simulink model "mariner_NNcont"  (R2018b)
settings: Solver=FixedStepAuto  StartTime=0.0  StopTime=600  FixedStep=0.1  RelTol=1e-3
libraries: neural x75, simulink x1
(part 3 of 3)

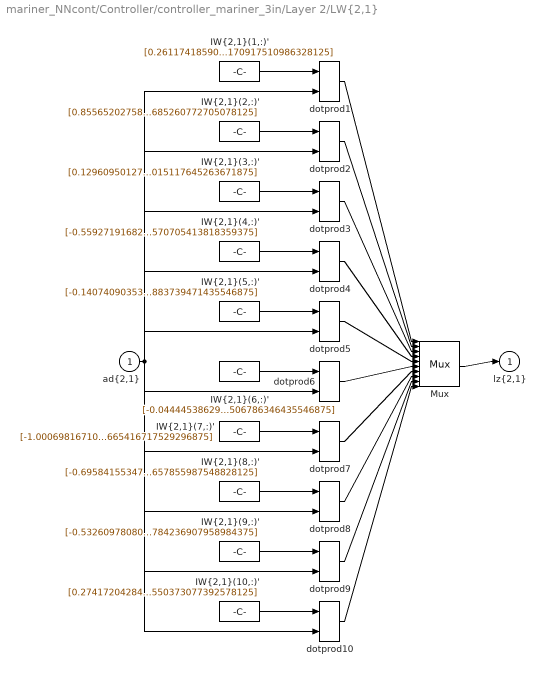
== system mariner_NNcont/Controller/controller_mariner_3in/Layer 2/LW{2,1} ==
  "ad{2,1}" : Inport  PortDimensions=10
      mask Display: e = 0.06;c1 = [120 230 180]/255;c2 = ([120 230 180]+0)/(256+128);c3 = ([120 230 180]+128)/(256+128);patch([0 1 1 0],[0 0 1 1],c1);patch([0 1 1 1-e 1-e 0+e],[0 0 1 1-e 0+e 0+e],c2);patch([0 0 1 1-e 0+e 0+e],[0 1 1 1-e 1-e 0+e],c3);plot([0 1 1 0 0],[0 0 1 1 0]);
  "IW{2,1}(1,:)'" : Constant  Value=[0.261174185904248068457178533208207227289676666259765625;-0.003283003051929162842414999801121666678227484226226806640625;0.21894073243983969145887158447294495999813079833984375;0.1719351505134853186351762133199372328817844390869140625;-0.79630547007300067630097828441648744046688079833984375;-0.444574661776908464094759665385936386883258819580078125;0.906078837819613180926126005942933261394500732421875;-0.5775547854832592253870870990795083343982696533203125;0.3749229122076920273087807800038717687129974365234375;-0.91313009543488476982275869886507280170917510986328125]
      mask Display: e = 0.06;c1 = [120 150 230]/255;c2 = ([120 150 230]+0)/383;c3 = ([120 150 230]+128)/383;patch([0 1 1 0],[0 0 1 1],c1);patch([0 1 1 1-e 1-e 0+e],[0 0 1 1-e 0+e 0+e],c2);patch([0 0 1 1-e 0+e 0+e],[0 1 1 1-e 1-e 0+e],c3);plot([0 1 1 0 0],[0 0 1 1 0]);disp('weights');
  "IW{2,1}(10,:)'" : Constant  Value=[0.2741720428489411442996015466633252799510955810546875;-0.331267567288568820504934819837217219173908233642578125;0.08501797064077308563323498447061865590512752532958984375;-0.13802843406108300516876852270797826349735260009765625;-0.66775067067659055197736961417831480503082275390625;0.65274589167754093477213928053970448672771453857421875;0.60325942316056535563717488912516273558139801025390625;0.76541902649870774411056117969565093517303466796875;-0.302998665532592859062077650378341786563396453857421875;1.014969024792983010030411605839617550373077392578125]
      mask Display: e = 0.06;c1 = [120 150 230]/255;c2 = ([120 150 230]+0)/383;c3 = ([120 150 230]+128)/383;patch([0 1 1 0],[0 0 1 1],c1);patch([0 1 1 1-e 1-e 0+e],[0 0 1 1-e 0+e 0+e],c2);patch([0 0 1 1-e 0+e 0+e],[0 1 1 1-e 1-e 0+e],c3);plot([0 1 1 0 0],[0 0 1 1 0]);disp('weights');
  "IW{2,1}(2,:)'" : Constant  Value=[0.85565202758614222755539913123357109725475311279296875;-0.283056952913707082775118806239333935081958770751953125;-0.2258338801321223832108131546192453242838382720947265625;0.77075660919109056923304024167009629309177398681640625;-0.1294753607797942962509551989569445140659809112548828125;0.152371280591739377552329415266285650432109832763671875;0.0399229534231867744242805429166764952242374420166015625;-0.75982138249167163746022879422525875270366668701171875;-0.80225466104966314251356607201159931719303131103515625;-0.62172867186234548331214000427280552685260772705078125]
      mask Display: e = 0.06;c1 = [120 150 230]/255;c2 = ([120 150 230]+0)/383;c3 = ([120 150 230]+128)/383;patch([0 1 1 0],[0 0 1 1],c1);patch([0 1 1 1-e 1-e 0+e],[0 0 1 1-e 0+e 0+e],c2);patch([0 0 1 1-e 0+e 0+e],[0 1 1 1-e 1-e 0+e],c3);plot([0 1 1 0 0],[0 0 1 1 0]);disp('weights');
  "IW{2,1}(3,:)'" : Constant  Value=[0.1296095012754385766839959615026600658893585205078125;-0.94480799299970896765188399513135664165019989013671875;-0.4301375963937488222654792480170726776123046875;0.459664837526012615143145012552849948406219482421875;0.1934938854259011520309030629505286924540996551513671875;0.303590659028730447399624381432658992707729339599609375;0.0250667137529580787147498455169625231064856052398681640625;-0.7718185476396290933820409918553195893764495849609375;-0.7919589744969688371867277965066023170948028564453125;-0.6689404878056404157860015402548015117645263671875]
      mask Display: e = 0.06;c1 = [120 150 230]/255;c2 = ([120 150 230]+0)/383;c3 = ([120 150 230]+128)/383;patch([0 1 1 0],[0 0 1 1],c1);patch([0 1 1 1-e 1-e 0+e],[0 0 1 1-e 0+e 0+e],c2);patch([0 0 1 1-e 0+e 0+e],[0 1 1 1-e 1-e 0+e],c3);plot([0 1 1 0 0],[0 0 1 1 0]);disp('weights');
  "IW{2,1}(4,:)'" : Constant  Value=[-0.5592719168271766960742752416990697383880615234375;-0.63972010553606384331004619525629095733165740966796875;0.86712354687803727681938426030683331191539764404296875;-0.60202632961644775289045128374709747731685638427734375;0.04675818126060522772480254616311867721378803253173828125;-0.6845715113228525439126315177418291568756103515625;0.1082908321127431239272453922239947132766246795654296875;-0.2114272144397531250081812004282255657017230987548828125;0.1653939942029022114322600600644364021718502044677734375;0.85845774340393798951254211715422570705413818359375]
      mask Display: e = 0.06;c1 = [120 150 230]/255;c2 = ([120 150 230]+0)/383;c3 = ([120 150 230]+128)/383;patch([0 1 1 0],[0 0 1 1],c1);patch([0 1 1 1-e 1-e 0+e],[0 0 1 1-e 0+e 0+e],c2);patch([0 0 1 1-e 0+e 0+e],[0 1 1 1-e 1-e 0+e],c3);plot([0 1 1 0 0],[0 0 1 1 0]);disp('weights');
  "IW{2,1}(5,:)'" : Constant  Value=[-0.14074090353561474753263382808654569089412689208984375;-0.1582177881605986990987133822272880934178829193115234375;0.76789061341721709386121119678136892616748809814453125;-0.64243771524855175503176951679051853716373443603515625;0.6982728307682517510102115920744836330413818359375;0.0301621836322126524176923112463555298745632171630859375;0.34029705620992156678283890869352035224437713623046875;0.771669895262477201214323940803296864032745361328125;0.430887484942656551201167758335941471159458160400390625;0.82439589529222967456689730170182883739471435546875]
      mask Display: e = 0.06;c1 = [120 150 230]/255;c2 = ([120 150 230]+0)/383;c3 = ([120 150 230]+128)/383;patch([0 1 1 0],[0 0 1 1],c1);patch([0 1 1 1-e 1-e 0+e],[0 0 1 1-e 0+e 0+e],c2);patch([0 0 1 1-e 0+e 0+e],[0 1 1 1-e 1-e 0+e],c3);plot([0 1 1 0 0],[0 0 1 1 0]);disp('weights');
  "IW{2,1}(6,:)'" : Constant  Value=[-0.04444538629282100694606327806468470953404903411865234375;0.1633126529035742457995894483246956951916217803955078125;0.93328352617765852894393674432649277150630950927734375;0.1312587739791350738283171040166052989661693572998046875;-0.88766423248751002983425451020593754947185516357421875;-0.00598139511896102205046332755955518223345279693603515625;-0.86611856253597918620101836495450697839260101318359375;-0.785777466061251761431094564613886177539825439453125;-0.10379331601532486295536017451013321988284587860107421875;-0.1520954521603174736110730691507342271506786346435546875]
      mask Display: e = 0.06;c1 = [120 150 230]/255;c2 = ([120 150 230]+0)/383;c3 = ([120 150 230]+128)/383;patch([0 1 1 0],[0 0 1 1],c1);patch([0 1 1 1-e 1-e 0+e],[0 0 1 1-e 0+e 0+e],c2);patch([0 0 1 1-e 0+e 0+e],[0 1 1 1-e 1-e 0+e],c3);plot([0 1 1 0 0],[0 0 1 1 0]);disp('weights');
  "IW{2,1}(7,:)'" : Constant  Value=[-1.0006981671063766015095097827725112438201904296875;0.60941030927903039327020451310090720653533935546875;-0.02375081956900626511952623332035727798938751220703125;-0.155539049648913241252756733956630341708660125732421875;-0.87176861100853397790189092120272107422351837158203125;0.2349462648057879798901836920776986517012119293212890625;-0.78217384326468419875055815282394178211688995361328125;-0.4284269793998471964613372620078735053539276123046875;-0.25720118636501931863591607907437719404697418212890625;0.17938257051239059336467107641510665416717529296875]
      mask Display: e = 0.06;c1 = [120 150 230]/255;c2 = ([120 150 230]+0)/383;c3 = ([120 150 230]+128)/383;patch([0 1 1 0],[0 0 1 1],c1);patch([0 1 1 1-e 1-e 0+e],[0 0 1 1-e 0+e 0+e],c2);patch([0 0 1 1-e 0+e 0+e],[0 1 1 1-e 1-e 0+e],c3);plot([0 1 1 0 0],[0 0 1 1 0]);disp('weights');
  "IW{2,1}(8,:)'" : Constant  Value=[-0.69584155347007980996210108060040511190891265869140625;0.75309159965000371794729971952619962394237518310546875;-0.75210268731275908837830002084956504404544830322265625;0.71218767580268649286523441332974471151828765869140625;0.69666567607896545677448330025072209537029266357421875;0.106029491219146565494924061567871831357479095458984375;0.293510496575862589452299289405345916748046875;-0.276039693004178798840797526281676255166530609130859375;-0.10816770394463266768969589293192257173359394073486328125;0.652295803383552641463438703794963657855987548828125]
      mask Display: e = 0.06;c1 = [120 150 230]/255;c2 = ([120 150 230]+0)/383;c3 = ([120 150 230]+128)/383;patch([0 1 1 0],[0 0 1 1],c1);patch([0 1 1 1-e 1-e 0+e],[0 0 1 1-e 0+e 0+e],c2);patch([0 0 1 1-e 0+e 0+e],[0 1 1 1-e 1-e 0+e],c3);plot([0 1 1 0 0],[0 0 1 1 0]);disp('weights');
  "IW{2,1}(9,:)'" : Constant  Value=[-0.53260978080398280187779391781077720224857330322265625;0.7797854193828011037936676075332798063755035400390625;1.0309904985328952609080488400650210678577423095703125;0.2090678564933573790884935306166880764067173004150390625;0.422970982361082270539753835691954009234905242919921875;-0.25386727615109305755680679794750176370143890380859375;0.64856644515765704550602777089807204902172088623046875;0.0214787671671146894458725995491477078758180141448974609375;0.402204635550879763261633570436970330774784088134765625;-0.53082955432786516070109428255818784236907958984375]
      mask Display: e = 0.06;c1 = [120 150 230]/255;c2 = ([120 150 230]+0)/383;c3 = ([120 150 230]+128)/383;patch([0 1 1 0],[0 0 1 1],c1);patch([0 1 1 1-e 1-e 0+e],[0 0 1 1-e 0+e 0+e],c2);patch([0 0 1 1-e 0+e 0+e],[0 1 1 1-e 1-e 0+e],c3);plot([0 1 1 0 0],[0 0 1 1 0]);disp('weights');
  Mux : Mux  Inputs=10
      mask Display: e = 0.06;c1 = [120 150 230]/255;c2 = ([120 150 230]+0)/383;c3 = ([120 150 230]+128)/383;patch([0 1 1 0],[0 0 1 1],c1);patch([0 1 1 1-e 1-e 0+e],[0 0 1 1-e 0+e 0+e],c2);patch([0 0 1 1-e 0+e 0+e],[0 1 1 1-e 1-e 0+e],c3);plot([0 1 1 0 0],[0 0 1 1 0]);disp('Mux');
  dotprod{1..10} (10 alike) : neural/Weight Functions/dotprod
  "lz{2,1}" : Outport
      mask Display: e = 0.06;c1 = [120 230 180]/255;c2 = ([120 230 180]+0)/(256+128);c3 = ([120 230 180]+128)/(256+128);patch([0 1 1 0],[0 0 1 1],c1);patch([0 1 1 1-e 1-e 0+e],[0 0 1 1-e 0+e 0+e],c2);patch([0 0 1 1-e 0+e 0+e],[0 1 1 1-e 1-e 0+e],c3);plot([0 1 1 0 0],[0 0 1 1 0]);
  wires:
  Mux/1 -> "lz{2,1}"/1
  dotprod10/1 -> Mux/10
  "IW{2,1}(10,:)'"/1 -> dotprod10/1
  dotprod9/1 -> Mux/9
  "IW{2,1}(9,:)'"/1 -> dotprod9/1
  dotprod8/1 -> Mux/8
  "IW{2,1}(8,:)'"/1 -> dotprod8/1
  dotprod7/1 -> Mux/7
  "IW{2,1}(7,:)'"/1 -> dotprod7/1
  dotprod6/1 -> Mux/6
  "IW{2,1}(6,:)'"/1 -> dotprod6/1
  dotprod5/1 -> Mux/5
  "IW{2,1}(5,:)'"/1 -> dotprod5/1
  dotprod4/1 -> Mux/4
  "IW{2,1}(4,:)'"/1 -> dotprod4/1
  dotprod3/1 -> Mux/3
  "IW{2,1}(3,:)'"/1 -> dotprod3/1
  dotprod2/1 -> Mux/2
  "IW{2,1}(2,:)'"/1 -> dotprod2/1
  dotprod1/1 -> Mux/1
  "ad{2,1}"/1 -> dotprod10/2, dotprod9/2, dotprod8/2, dotprod7/2, dotprod6/2, dotprod5/2, dotprod4/2, dotprod3/2, dotprod2/2, dotprod1/2
  "IW{2,1}(1,:)'"/1 -> dotprod1/1

== system mariner_NNcont/Controller/controller_mariner_3in/Layer 3/Delays 1 ==
  "p{3}" : Inport  PortDimensions=10
      mask Display: e = 0.06;c1 = [120 230 180]/255;c2 = ([120 230 180]+0)/(256+128);c3 = ([120 230 180]+128)/(256+128);patch([0 1 1 0],[0 0 1 1],c1);patch([0 1 1 1-e 1-e 0+e],[0 0 1 1-e 0+e 0+e],c2);patch([0 0 1 1-e 0+e 0+e],[0 1 1 1-e 1-e 0+e],c3);plot([0 1 1 0 0],[0 0 1 1 0]);
  mux : Mux  Inputs=1
      mask Display: e = 0.06;c1 = [120 150 230]/255;c2 = ([120 150 230]+0)/383;c3 = ([120 150 230]+128)/383;patch([0 1 1 0],[0 0 1 1],c1);patch([0 1 1 1-e 1-e 0+e],[0 0 1 1-e 0+e 0+e],c2);patch([0 0 1 1-e 0+e 0+e],[0 1 1 1-e 1-e 0+e],c3);plot([0 1 1 0 0],[0 0 1 1 0]);disp('Mux')
  "pd{3,2}" : Outport
      mask Display: e = 0.06;c1 = [120 230 180]/255;c2 = ([120 230 180]+0)/(256+128);c3 = ([120 230 180]+128)/(256+128);patch([0 1 1 0],[0 0 1 1],c1);patch([0 1 1 1-e 1-e 0+e],[0 0 1 1-e 0+e 0+e],c2);patch([0 0 1 1-e 0+e 0+e],[0 1 1 1-e 1-e 0+e],c3);plot([0 1 1 0 0],[0 0 1 1 0]);
  wires:
  mux/1 -> "pd{3,2}"/1
  "p{3}"/1 -> mux/1

== system mariner_NNcont/Controller/controller_mariner_3in/Layer 3/LW{3,2} ==
  "ad{3,2}" : Inport  PortDimensions=10
      mask Display: e = 0.06;c1 = [120 230 180]/255;c2 = ([120 230 180]+0)/(256+128);c3 = ([120 230 180]+128)/(256+128);patch([0 1 1 0],[0 0 1 1],c1);patch([0 1 1 1-e 1-e 0+e],[0 0 1 1-e 0+e 0+e],c2);patch([0 0 1 1-e 0+e 0+e],[0 1 1 1-e 1-e 0+e],c3);plot([0 1 1 0 0],[0 0 1 1 0]);
  "IW{3,2}(1,:)'" : Constant  Value=[0;0;0;-0.219212418107098738762061884699505753815174102783203125;-0.07583323193546000207110324708992266096174716949462890625;0;0;0.301667338509124915990611270899535156786441802978515625;0;-0.1456684791332186479362320596919744275510311126708984375]
      mask Display: e = 0.06;c1 = [120 150 230]/255;c2 = ([120 150 230]+0)/383;c3 = ([120 150 230]+128)/383;patch([0 1 1 0],[0 0 1 1],c1);patch([0 1 1 1-e 1-e 0+e],[0 0 1 1-e 0+e 0+e],c2);patch([0 0 1 1-e 0+e 0+e],[0 1 1 1-e 1-e 0+e],c3);plot([0 1 1 0 0],[0 0 1 1 0]);disp('weights');
  Mux : Mux  Inputs=1
      mask Display: e = 0.06;c1 = [120 150 230]/255;c2 = ([120 150 230]+0)/383;c3 = ([120 150 230]+128)/383;patch([0 1 1 0],[0 0 1 1],c1);patch([0 1 1 1-e 1-e 0+e],[0 0 1 1-e 0+e 0+e],c2);patch([0 0 1 1-e 0+e 0+e],[0 1 1 1-e 1-e 0+e],c3);plot([0 1 1 0 0],[0 0 1 1 0]);disp('Mux');
  dotprod1 : neural/Weight Functions/dotprod
  "lz{3,2}" : Outport
      mask Display: e = 0.06;c1 = [120 230 180]/255;c2 = ([120 230 180]+0)/(256+128);c3 = ([120 230 180]+128)/(256+128);patch([0 1 1 0],[0 0 1 1],c1);patch([0 1 1 1-e 1-e 0+e],[0 0 1 1-e 0+e 0+e],c2);patch([0 0 1 1-e 0+e 0+e],[0 1 1 1-e 1-e 0+e],c3);plot([0 1 1 0 0],[0 0 1 1 0]);
  wires:
  Mux/1 -> "lz{3,2}"/1
  dotprod1/1 -> Mux/1
  "ad{3,2}"/1 -> dotprod1/2
  "IW{3,2}(1,:)'"/1 -> dotprod1/1

== matlab function mariner_NNcont/MATLAB Function1 ==
  data: xdot input; xnext output; x input; h input
function xnext = euler2(xdot,x,h)
% EULER2  Integrate a system of ordinary differential equations using 
%	  Euler's 2nd-order method.
%
% xnext = euler2(xdot,x,h)
%
% xdot  - dx/dt(k) = f(x(k)
% x     - x(k)
% xnext - x(k+1)
% h     - step size
%
% Author:   Thor I. Fossen
% Date:     14th June 2001
% Revisions: 

xnext = x + h*xdot;

== matlab function mariner_NNcont/MATLAB Function ==
  data: x input; xdot output; ui input
function xdot   = mariner(x,ui)
% [xdot,U] = mariner(x,ui) returns the speed U in m/s (optionally) and the 
% time derivative of the state vector: x = [ u v r x y psi delta n ]'  for
% the Mariner class vessel L = 160.93 m, where
%
% u     = pertubed surge velocity about Uo (m/s)
% v     = pertubed sway velocity about zero (m/s)
% r     = pertubed yaw velocity about zero (rad/s)
% x     = position in x-direction (m)
% y     = position in y-direction (m)
% psi   = pertubed yaw angle about zero (rad)
% delta = actual rudder angle (rad)
%
% The inputs are :
% 
% ui    = commanded rudder angle (rad)
% U0    = nominal speed (optionally). Default value is U0 = 7.7175 m/s = 15 knots.
%
% Reference: M.S. Chislett and J. Stroem-Tejsen (1965). Planar Motion Mechanism Tests 
%            and Full-Scale Steering and Maneuvering Predictions for a Mariner Class Vessel,
%            Technical Report Hy-5, Hydro- and Aerodynamics Laboratory, Lyngby, Denmark.
% 
% Author:    Trygve Lauvdal
% Date:      12th May 1994
% Revisions: 19th July 2001 (Thor I. Fossen): added input/ouput U0 and U, changed order of x-vector
%            20th July 2001 (Thor I. Fossen): replaced inertia matrix with correct values
%            11th July 2003 (Thor I. Fossen): max rudder is changed from 30 deg to 40
%                            deg to satisfy IMO regulations for 35 deg rudder execute

% Check of input and state dimensions
if (length(x)  ~= 7),error('x-vector must have dimension 7 !'); end
if (length(ui) ~= 1),error('ui must be a scalar input!'); end
%if nargin==2, U0 = 7.7175; end

U0 = 7.7175;

% Normalization variables
L = 160.93;
U = sqrt((U0 + x(1))^2 + x(2)^2);

% Non-dimensional states and inputs
delta_c = -ui;   % delta_c = -ui such that positive delta_c -> positive r

u     = x(1)/U;   
v     = x(2)/U;  
r     = x(3)*L/U; 
psi   = x(6); 
delta = x(7); 

% Parameters, hydrodynamic derivatives and main dimensions
delta_max  = 40;           % max rudder angle      (deg)
Ddelta_max = 5;            % max rudder derivative (deg/s)

m  = 798e-5;
Iz = 39.2e-5;
xG = -0.023;

Xudot =  -42e-5;   Yvdot =  -748e-5;   Nvdot = 4.646e-5;
Xu    = -184e-5;   Yrdot =-9.354e-5;   Nrdot = -43.8e-5;
Xuu   = -110e-5;   Yv    = -1160e-5;   Nv    =  -264e-5;
Xuuu  = -215e-5;   Yr    =  -499e-5;   Nr    =  -166e-5;
Xvv   = -899e-5;   Yvvv  = -8078e-5;   Nvvv  =  1636e-5;
Xrr   =   18e-5;   Yvvr  = 15356e-5;   Nvvr  = -5483e-5;
Xdd   =  -95e-5;   Yvu   = -1160e-5;   Nvu   =  -264e-5;
Xudd  = -190e-5;   Yru   =  -499e-5;   Nru   =  -166e-5;
Xrv   =  798e-5;   Yd    =   278e-5;   Nd    =  -139e-5;
Xvd   =   93e-5;   Yddd  =   -90e-5;   Nddd  =    45e-5;
Xuvd  =   93e-5;   Yud   =   556e-5;   Nud   =  -278e-5;
                   Yuud  =   278e-5;   Nuud  =  -139e-5;
                   Yvdd  =    -4e-5;   Nvdd  =    13e-5;
                   Yvvd  =  1190e-5;   Nvvd  =  -489e-5;
                   Y0    =    -4e-5;   N0    =     3e-5;
                   Y0u   =    -8e-5;   N0u   =     6e-5;
                   Y0uu  =    -4e-5;   N0uu  =     3e-5;

% Masses and moments of inertia
m11 = m-Xudot;
m22 = m-Yvdot;
m23 = m*xG-Yrdot;
m32 = m*xG-Nvdot;
m33 = Iz-Nrdot;

% Rudder saturation and dynamics
if abs(delta_c) >= delta_max*pi/180,
   delta_c = sign(delta_c)*delta_max*pi/180;
end
delta_dot = delta_c - delta;
if abs(delta_dot) >= Ddelta_max*pi/180,
   delta_dot = sign(delta_dot)*Ddelta_max*pi/180;
end

% Forces and moments
X = Xu*u + Xuu*u^2 + Xuuu*u^3 + Xvv*v^2 + Xrr*r^2 + Xrv*r*v + Xdd*delta^2 +...
    Xudd*u*delta^2 + Xvd*v*delta + Xuvd*u*v*delta;

Y = Yv*v + Yr*r + Yvvv*v^3 + Yvvr*v^2*r + Yvu*v*u + Yru*r*u + Yd*delta + ...
    Yddd*delta^3 + Yud*u*delta + Yuud*u^2*delta + Yvdd*v*delta^2 + ...
    Yvvd*v^2*delta + (Y0 + Y0u*u + Y0uu*u^2);

N = Nv*v + Nr*r + Nvvv*v^3 + Nvvr*v^2*r + Nvu*v*u + Nru*r*u + Nd*delta + ...
    Nddd*delta^3 + Nud*u*delta + Nuud*u^2*delta + Nvdd*v*delta^2 + ...
    Nvvd*v^2*delta + (N0 + N0u*u + N0uu*u^2);

% Dimensional state derivative
detM22 = m22*m33-m23*m32;

xdot = [           X*(U^2/L)/m11
        -(-m33*Y+m23*N)*(U^2/L)/detM22
         (-m32*Y+m22*N)*(U^2/L^2)/detM22
           (cos(psi)*(U0/U+u)-sin(psi)*v)*U
           (sin(psi)*(U0/U+u)+cos(psi)*v)*U  
                    r*(U/L)
                    delta_dot                  ];

== stateflow chart mariner_NNcont/mariner ==
  settings: updateMethod=CONTINUOUS
  state mariner
    %% initialize values when entry
    en:
    L = 160.93;
    m = 798*10^-5;
    xG = -0.023;
    Iz = 39.2*10^-5;
    Xudot =  -42e-5;  Yvdot =  -748e-5;  Nvdot = 4.646e-5;
    Xu  = -184e-5;   Yrdot =-9.354e-5;   Nrdot = -43.8e-5;
    Xuu = -110e-5;   Yv = -1160e-5;   Nv =  -264e-5;
    Xuuu = -215e-5;   Yr =  -499e-5;   Nr =  -166e-5;
    Xvv = -899e-5;   Yvvv = -8078e-5;   Nvvv =  1636e-5;
    Xrr =   18e-5;   Yvvr = 15356e-5;   Nvvr = -5483e-5;
    Xdd =  -95e-5;   Yvu = -1160e-5;   Nvu =  -264e-5;
    Xudd = -190e-5;   Yru =  -499e-5;   Nru =  -166e-5;
    Xrv =  798e-5;   Yd  =   278e-5;   Nd =  -139e-5;
    Xvd =   93e-5;   Yddd  =   -90e-5;   Nddd =    45e-5;
    Xuvd =   93e-5;   Yud = 556e-5;   Nud =  -278e-5;
    Yuud =   278e-5;   Nuud  =  -139e-5;
    Yvdd  =    -4e-5;   Nvdd  = 13e-5;
    Yvvd  =  1190e-5;   Nvvd  = -489e-5;
    Y0 = -4e-5;   N0 =  3e-5;
    Y0u  =  -8e-5;   N0u = 6e-5;
    Y0uu =  -4e-5;   N0uu  =  3e-5;
    m11 = 798*10^-5 - (-42e-5);
    m22 = 798*10^-5 - ( -748e-5);
    m23 = 798*10^-5 * -0.023 - (-9.354e-5);
    m32 = 798*10^-5 * -0.023 - 4.646e-5;
    m33 = 39.2*10^-5 -  (-43.8e-5);
    %detM22 = m22*m33-m23*m32;
    %detM22 = ((798*10^-5 - ( -748e-5))*(39.2*10^-5 -  (-43.8e-5)) - (798*10^-5 * -0.023 - (-9.354e-5))*(798*10^-5 * -0.023 - 4.646e-5));
    delta_max = 40;
    Ddelta_max = 5;
    % u
    %Executing updates of system during simulation
    du:
    %delta_c = min(max(-ui,-delta_max*pi/180),delta_max*pi/180) ;
    %U = (sqrt((ui + u)^2 + v^2));
    %delta_do = (-ui - delta);
    %X = Xu*u/(sqrt((ui + u)^2 + v^2)) + Xuu*(u/(sqrt((ui + u)^2 + v^2)))^2 + Xuuu*(u/(sqrt((ui + u)^2 + v^2)))^3 + Xvv*(v/(sqrt((ui + u)^2 + v^2)))^2 + Xrr*(r*L/(sqrt((ui + u)^2 + v^2)))^2 + Xrv*(r*L/(sqrt((ui + u)^2 + v^2)))*(v/(sqrt((ui + u)^2 + v^2))) + Xdd*delta^2 +Xudd*(u/(sqrt((ui + u)^2 + v^2)))*delta^2 + Xvd*(v/(sqrt((ui + u)^2 + v^2)))*delta + Xuvd*(u/(sqrt((ui + u)^2 + v^2)))*(v/(sqrt((ui + u)^2 + v^2)))*delta;
    %Y = Yv*v + Yr*r + Yvvv*v^3 + Yvvr*v^2*r + Yvu*v*u + Yru*r*u + Yd*delta + Yddd*delta^3 + Yud*u*delta + Yuud*u^2*delta + Yvdd*v*delta^2 + Yvvd*v^2*delta + (Y0 + Y0u*u + Y0uu*u^2);
    %N = Nv*v + Nr*r + Nvvv*v^3 + Nvvr*v^2*r + Nvu*v*u + Nru*r*u + Nd*delta + Nddd*delta^3 + Nud*u*delta + Nuud*u^2*delta + Nvdd*v*delta^2 + Nvvd*v^2*delta + (N0 + N0u*u + N0uu*u^2);
    u_dot = (Xu*(u/(sqrt((ui + u)^2 + v^2))) + Xuu*(u/(sqrt((ui + u)^2 + v^2)))^2 + Xuuu*(u/(sqrt((ui + u)^2 + v^2)))^3 + Xvv*(v/(sqrt((ui + u)^2 + v^2)))^2 + Xrr*(r*L/(sqrt((ui + u)^2 + v^2)))^2 + Xrv*(r*L/(sqrt((ui + u)^2 + v^2)))*(v/(sqrt((ui + u)^2 + v^2))) + Xdd*delta^2 +Xudd*(u/(sqrt((ui + u)^2 + v^2)))*delta^2 + Xvd*(v/(sqrt((ui + u)^2 + v^2)))*delta + Xuvd*(u/(sqrt((ui + u)^2 + v^2)))*(v/(sqrt((ui + u)^2 + v^2)))*delta)*((sqrt((ui + u)^2 + v^2))^2 /L)/(798*10^-5 - (-42e-5));
    v_dot =  -(-(39.2*10^-5 -  (-43.8e-5))*(Yv*(v/(sqrt((ui + u)^2 + v^2))) + Yr*(r*L/(sqrt((ui + u)^2 + v^2))) + Yvvv*(v/(sqrt((ui + u)^2 + v^2)))^3 + Yvvr*(v/(sqrt((ui + u)^2 + v^2)))^2 * (r*L/(sqrt((ui + u)^2 + v^2))) + Yvu*(v/(sqrt((ui + u)^2 + v^2)))*(u/(sqrt((ui + u)^2 + v^2))) + Yru*(r*L/(sqrt((ui + u)^2 + v^2)))*(u/(sqrt((ui + u)^2 + v^2))) + Yd*delta + Yddd*delta^3 + Yud*(u/(sqrt((ui + u)^2 + v^2)))*delta + Yuud*(u/(sqrt((ui + u)^2 + v^2)))^2*delta + Yvdd*(v/(sqrt((ui + u)^2 + v^2)))*delta^2 + Yvvd*(v/(sqrt((ui + u)^2 + v^2)))^2*delta + (Y0 + Y0u*(u/(sqrt((ui + u)^2 + v^2))) + Y0uu*(u/(sqrt((ui + u)^2 + v^2)))^2))+(798*10^-5 * -0.023 - (-9.354e-5))*(Nv*(v/(sqrt((ui + u)^2 + v^2))) + Nr*(r*L/(sqrt((ui + u)^2 + v^2))) + Nvvv*(v/(sqrt((ui + u)^2 + v^2)))^3 + Nvvr*(v/(sqrt((ui + u)^2 + v^2)))^2*(r*L/(sqrt((ui + u)^2 + v^2))) + Nvu*(v/(sqrt((ui + u)^2 + v^2)))*(u/(sqrt((ui + u)^2 + v^2))) + Nru*(r*L/(sqrt((ui + u)^2 + v^2)))*(u/(sqrt((ui + u)^2 + v^2))) + Nd*delta + Nddd*delta^3 + Nud*(u/(sqrt((ui + u)^2 + v^2)))*delta + Nuud*(u/(sqrt((ui + u)^2 + v^2)))^2*delta + Nvdd*(v/(sqrt((ui + u)^2 + v^2)))*delta^2 + Nvvd*v^2*delta + (N0 + N0u*u + N0uu*u^2)))*((sqrt((ui + u)^2 + v^2))^2/L)/((798*10^-5 - ( -748e-5))*(39.2*10^-5 -  (-43.8e-5)) - (798*10^-5 * -0.023 - (-9.354e-5))*(798*10^-5 * -0.023 - 4.646e-5)) ;
    r_dot = (-(798*10^-5 * -0.023 - 4.646e-5)*(Yv*(v/(sqrt((ui + u)^2 + v^2))) + Yr*(r*L/(sqrt((ui + u)^2 + v^2))) + Yvvv*(v/(sqrt((ui + u)^2 + v^2)))^3 + Yvvr*(v/(sqrt((ui + u)^2 + v^2)))^2*(r*L/(sqrt((ui + u)^2 + v^2))) + Yvu*(v/(sqrt((ui + u)^2 + v^2)))*(u/(sqrt((ui + u)^2 + v^2))) + Yru*(r*L/(sqrt((ui + u)^2 + v^2)))*(u/(sqrt((ui + u)^2 + v^2))) + Yd*delta + Yddd*delta^3 + Yud*(u/(sqrt((ui + u)^2 + v^2)))*delta + Yuud*(u/(sqrt((ui + u)^2 + v^2)))^2*delta + Yvdd*(v/(sqrt((ui + u)^2 + v^2)))*delta^2 + Yvvd*(v/(sqrt((ui + u)^2 + v^2)))^2*delta + (Y0 + Y0u*(u/(sqrt((ui + u)^2 + v^2))) + Y0uu*(u/(sqrt((ui + u)^2 + v^2)))^2))+(798*10^-5 - ( -748e-5))*(Nv*(v/(sqrt((ui + u)^2 + v^2))) + Nr*(r*L/(sqrt((ui + u)^2 + v^2))) + Nvvv*(v/(sqrt((ui + u)^2 + v^2)))^3 + Nvvr*(v/(sqrt((ui + u)^2 + v^2)))^2*(r*L/(sqrt((ui + u)^2 + v^2))) + Nvu*(v/(sqrt((ui + u)^2 + v^2)))*(u/(sqrt((ui + u)^2 + v^2))) + Nru*(r*L/(sqrt((ui + u)^2 + v^2)))*(u/(sqrt((ui + u)^2 + v^2))) + Nd*delta + Nddd*delta^3 + Nud*(u/(sqrt((ui + u)^2 + v^2)))*delta + Nuud*(u/(sqrt((ui + u)^2 + v^2)))^2*delta + Nvdd*(v/(sqrt((ui + u)^2 + v^2)))*delta^2 + Nvvd*(v/(sqrt((ui + u)^2 + v^2)))^2*delta + (N0 + N0u*(u/(sqrt((ui + u)^2 + v^2))) + N0uu*(u/(sqrt((ui + u)^2 + v^2)))^2)))*((sqrt((ui + u)^2 + v^2))^2/L^2)/((798*10^-5 - ( -748e-5))*(39.2*10^-5 -  (-43.8e-5)) - (798*10^-5 * -0.023 - (-9.354e-5))*(798*10^-5 * -0.023 - 4.646e-5)) ;
    x_dot = (cos(psi)*(U0/(sqrt((ui + u)^2 + v^2))+(u/(sqrt((ui + u)^2 + v^2))))-sin(psi)*(v/(sqrt((ui + u)^2 + v^2))))*(sqrt((ui + u)^2 + v^2)) ;
    y_dot = (sin(psi)*(U0/(sqrt((ui + u)^2 + v^2))+(u/(sqrt((ui + u)^2 + v^2))))+cos(psi)*(v/(sqrt((ui + u)^2 + v^2))))*(sqrt((ui + u)^2 + v^2)) ;
    psi_dot = (r*L/(sqrt((ui + u)^2 + v^2)))*((sqrt((ui + u)^2 + v^2))/L);
    delta_dot = min(max(((min(max(-ui,-delta_max*pi/180),delta_max*pi/180)) - delta),-Ddelta_max*pi/180),Ddelta_max*pi/180) ;
    %% OUTPUTS
    u_out = u;
    v_out = v;
    r_out = r;
    x_out = x;
    y_out = y;
    psi_out = psi;
    delta_out = delta;
  (default) -> ? [order 1]
  (default) -> mariner [order 1] : {u = 0.01;
      | v = 0.01;
      | r = 0.01;
      | x = 0.01;
      | y = 0.01;
      | psi = 0.01;
      | delta = 0.01;}
  data: u_out output; v_out output; u local; ui input; v local; Nvdot local double; Iz local double; L local double; Yvdot local double; xG local double; m local double; Xudot local double; Xuu local double; Yv local double; Xuuu local double; Nrdot local double; Nv local double; Yr local double; Yrdot local double; Xu local double; Nr local double; Xrr local double; Xdd local double; Yvvv local double; Yvu local double; Nvvv local double; Yvvr local double; Nvvr local double; Xvv local double; Xvd local double; Yru local double; Nd local double; Nvu local double; Xudd local double; Nru local double; Yd local double; Xrv local double; Nvdd local double; Yud local double; Yuud local double; Xuvd local double; Yvdd local double; Nud local double; Nuud local double; Yddd local double; Nddd local double; Y0uu local double; N0uu local double; N0 local double; N0u local double; Y0 local double; Yvvd local double; Nvvd local double; Y0u local double; m11 local double; m32 local double; m22 local double; m23 local double; m33 local double; U0 input; r_out output; r local; psi local; x local; y local; delta local; Ddelta_max local double; delta_max local double; N local double; x_out output; y_out output; psi_out output double; delta_out output
  data u settings: updateMethod=SF_CONTINUOUS_TIME_DATA
  data v settings: updateMethod=SF_CONTINUOUS_TIME_DATA
  data r settings: updateMethod=SF_CONTINUOUS_TIME_DATA
  data psi settings: updateMethod=SF_CONTINUOUS_TIME_DATA
  data x settings: updateMethod=SF_CONTINUOUS_TIME_DATA
  data y settings: updateMethod=SF_CONTINUOUS_TIME_DATA
  data delta settings: updateMethod=SF_CONTINUOUS_TIME_DATA

== matlab function mariner_NNcont/Controller/Normalize ==
  data: u input; y output
function y = fcn(u)
max_r = 0.0029; min_r = -4.9078e-04;
max_psi = 0.1295; min_psi = 0;
y = zeros(3,1);
y(1) = (u(1) -min_r)/(max_r - min_r);% r
y(2) = (u(2) -min_psi)/(max_psi - min_psi);
y(3) = u(3);

== matlab function mariner_NNcont/Controller/denormalize ==
  data: u input; y output
function y = fcn(u)
max_delta = 0.0445; min_delta = -0.0779;
y = zeros(1,1);
y(1) = u(1)*(max_delta - min_delta)+min_delta;% r
